simulink model "freq_testing"  (R2018b)
settings: Solver=VariableStepAuto  StartTime=0.0  StopTime=10.0  RelTol=1e-3
libraries: simulink x3, cf_lib x1, vel_controller_lib x1
settings Model: Creator=Pontus  LastModifiedBy=Pontus

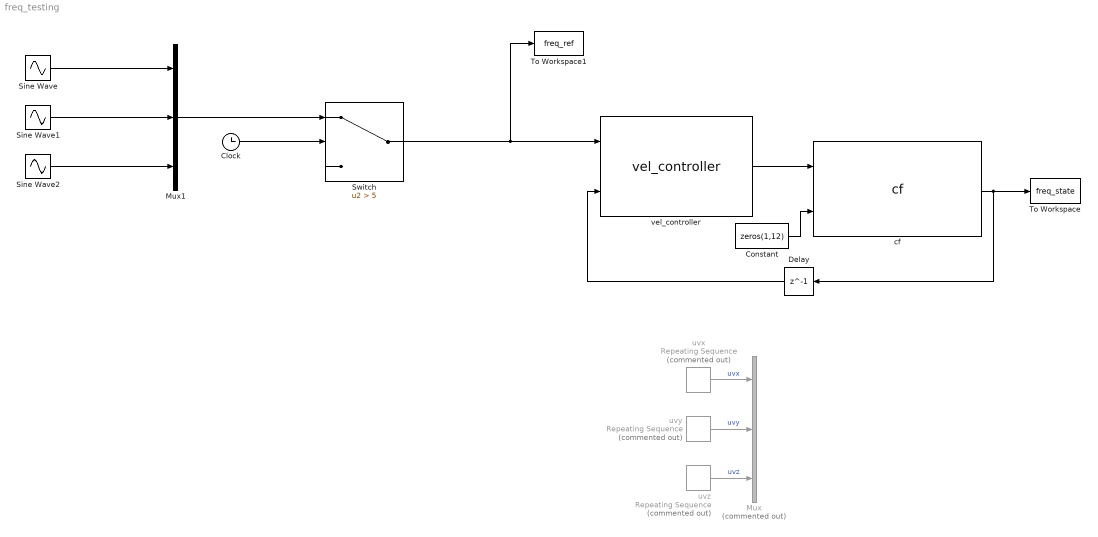
== system freq_testing ==
  Clock : Clock
      settings: Decimation=100
  Constant : Constant  Value=zeros(1,12)
  Delay : Delay  DelayLength=1
  Mux : Mux  Commented=on  Inputs=3
  Mux1 : Mux  Inputs=3
  Sine Wave : Sin  SampleTime=0
  Sine Wave1 : Sin  SampleTime=0
  Sine Wave2 : Sin  SampleTime=0
  Switch : Switch  Criteria=u2 > Threshold  Threshold=5
  To Workspace : ToWorkspace  VariableName=freq_state  SaveFormat=Timeseries  SampleTime=-1
  To Workspace1 : ToWorkspace  VariableName=freq_ref  SaveFormat=Timeseries  SampleTime=-1
  cf : cf_lib/cf  SystemSampleTime=-1
  uvx : simulink/Sources/Repeating Sequence  Commented=on  rep_seq_t=[0 2].'  rep_seq_y=ref.x
  uvy : simulink/Sources/Repeating Sequence  Commented=on  rep_seq_t=[0 5].'  rep_seq_y=ref.y
  uvz : simulink/Sources/Repeating Sequence  Commented=on  rep_seq_t=time_ref  rep_seq_y=ref.z
  vel_controller : vel_controller_lib/vel_controller  SystemSampleTime=-1
  wires:
  uvz/1 -> Mux/3  "uvz"
  uvy/1 -> Mux/2  "uvy"
  Delay/1 -> vel_controller/2
  vel_controller/1 -> cf/1
  cf/1 -> To Workspace/1, Delay/1
  Constant/1 -> cf/2
  uvx/1 -> Mux/1  "uvx"
  Sine Wave2/1 -> Mux1/3
  Sine Wave1/1 -> Mux1/2
  Sine Wave/1 -> Mux1/1
  Switch/1 -> To Workspace1/1, vel_controller/1
  Mux1/1 -> Switch/1
  Clock/1 -> Switch/2
